simulink model "Tak11_2"  (R2021a)
settings: Solver=VariableStepAuto  StartTime=0.0  StopTime=5  RelTol=1e-3
values from neighbouring files (symbols this model uses):
  A = [5 3 ... (first row only)    [T_5.m]
  B = [0 ... (first row only)    [T_5.m]
  B_f = [4 ... (first row only)    [T_5.m]
  C = [5 0]    [T_5.m]
  D = 6    [T_5.m]
  Gamma_f = [0 1 ... (first row only)    [T_5.m]
  H_f = [1 0]    [T_5.m]
  K = -H/M    [T_5.m]
  Lf = double([s.lf1 s.lf2])    [T_5.m]
  xif_0 = double([xi_f_1(0); xi_f_2(0)])    [T_5.m]
settings Model: Creator=fedor  LastModifiedBy=fedor

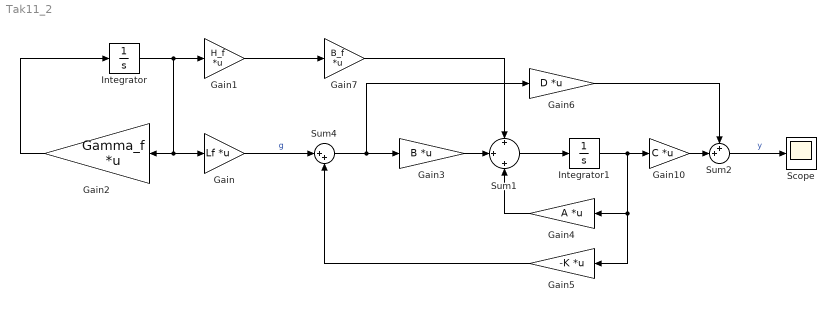
== system Tak11_2 ==
  Gain : Gain  Gain=Lf  Multiplication=Matrix(K*u)
  Gain1 : Gain  Gain=H_f  Multiplication=Matrix(K*u)
  Gain10 : Gain  Gain=C  Multiplication=Matrix(K*u)
  Gain2 : Gain  Gain=Gamma_f  Multiplication=Matrix(K*u)
  Gain3 : Gain  Gain=B  Multiplication=Matrix(K*u)
  Gain4 : Gain  Gain=A  Multiplication=Matrix(K*u)
  Gain5 : Gain  Gain=-K  Multiplication=Matrix(K*u)
  Gain6 : Gain  Gain=D  Multiplication=Matrix(K*u)
  Gain7 : Gain  Gain=B_f  Multiplication=Matrix(K*u)
  Integrator : Integrator  InitialCondition=xif_0
  Integrator1 : Integrator
  Scope : Scope
  Sum1 : Sum  Inputs=+|+|+
  Sum2 : Sum  Inputs=++|
  Sum4 : Sum  Inputs=|++
  wires:
  Gain2/1 -> Integrator/1
  Integrator/1 -> Gain1/1, Gain2/1, Gain/1
  Sum4/1 -> Gain6/1, Gain3/1
  Sum1/1 -> Integrator1/1
  Gain5/1 -> Sum4/2
  Gain4/1 -> Sum1/3
  Integrator1/1 -> Gain10/1, Gain4/1, Gain5/1
  Gain6/1 -> Sum2/1
  Gain/1 -> Sum4/1  "g"
  Gain10/1 -> Sum2/2
  Gain3/1 -> Sum1/2
  Gain7/1 -> Sum1/1
  Gain1/1 -> Gain7/1
  Sum2/1 -> Scope/1  "y"
